simulink model "transferencias_simu"  (R2021a)
settings: Solver=VariableStepAuto  StartTime=0.0  StopTime=20  RelTol=1e-3
settings Model: Creator=Santiago  LastModifiedBy=Santiago

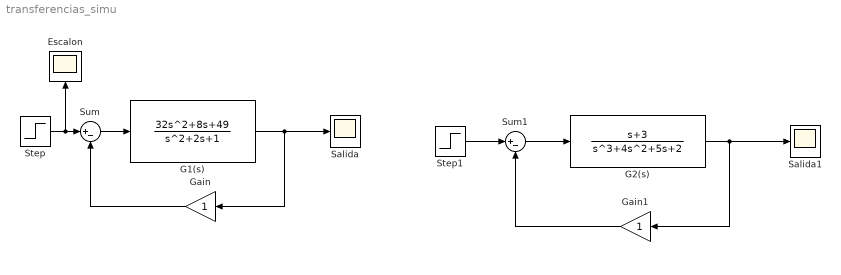
== system transferencias_simu ==
  Escalon : Scope
  G1(s) : TransferFcn  Numerator=[32 8 49]  ParameterTunability=Unconstrained
  G2(s) : TransferFcn  Numerator=[1 3]  Denominator=[1 4 5 2]
  Gain : Gain
  Gain1 : Gain
  Salida : Scope
  Salida1 : Scope
  Step : Step  SampleTime=0
  Step1 : Step  SampleTime=0
  Sum : Sum  Inputs=|+-
  Sum1 : Sum  Inputs=|+-
  wires:
  G1(s)/1 -> Salida/1, Gain/1
  Step/1 -> Escalon/1, Sum/1
  Gain/1 -> Sum/2
  Sum/1 -> G1(s)/1
  G2(s)/1 -> Salida1/1, Gain1/1
  Sum1/1 -> G2(s)/1
  Gain1/1 -> Sum1/2
  Step1/1 -> Sum1/1
